simulink model "lab3_e1"  (R2016a)
settings: Solver=VariableStepAuto  StartTime=0.0  StopTime=50  RelTol=1e-3
values from neighbouring files (symbols this model uses):
  C_D = H'    [lab3_sumup.m]
  G_D = G'    [lab3_sumup.m]
  H_D = C'    [lab3_sumup.m]
  L_db = acker(G_D, H_D, [p0, p1])    [lab3_sumup.m]
  L_ndb = acker(G_D, H_D, [p0, p1])    [lab3_sumup.m]
  Ts = 0.75    [lab3_sumup.m]
  x = [0 0.3]'    [lab3_sumup.m]
settings Model: Creator=Helvins  LastModifiedBy=Helvins

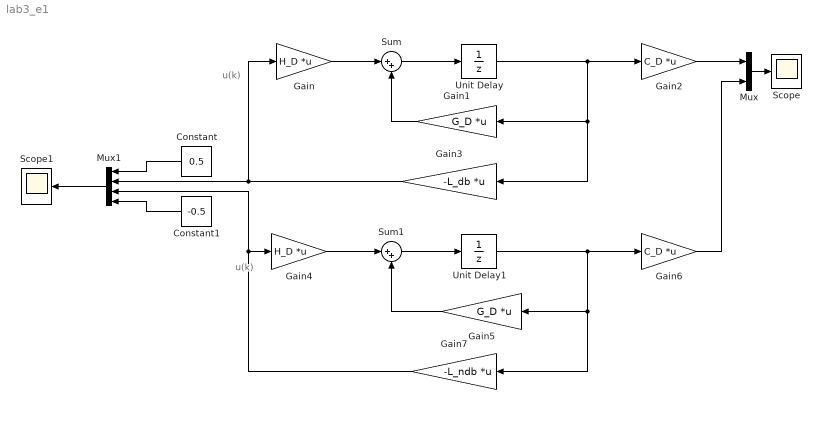
== system lab3_e1 ==
  note: u(k)
  note: u(k)
  Constant : Constant  Value=0.5
  Constant1 : Constant  Value=-0.5
  Gain : Gain  Gain=H_D  Multiplication=Matrix(K*u)
  Gain1 : Gain  Gain=G_D  Multiplication=Matrix(K*u)
  Gain2 : Gain  Gain=C_D  Multiplication=Matrix(K*u)
  Gain3 : Gain  Gain=-L_db  Multiplication=Matrix(K*u)
  Gain4 : Gain  Gain=H_D  Multiplication=Matrix(K*u)
  Gain5 : Gain  Gain=G_D  Multiplication=Matrix(K*u)
  Gain6 : Gain  Gain=C_D  Multiplication=Matrix(K*u)
  Gain7 : Gain  Gain=-L_ndb  Multiplication=Matrix(K*u)
  Mux : Mux  Inputs=2
  Mux1 : Mux
  Scope : Scope
  Scope1 : Scope
  Sum : Sum  Inputs=|++
  Sum1 : Sum  Inputs=|++
  Unit Delay : UnitDelay  InitialCondition=[x(1);x(2)]  SampleTime=Ts
  Unit Delay1 : UnitDelay  InitialCondition=[x(1);x(2)]  SampleTime=Ts
  wires:
  Gain/1 -> Sum/1
  Gain1/1 -> Sum/2
  Sum/1 -> Unit Delay/1
  Unit Delay/1 -> Gain1/1, Gain3/1, Gain2/1
  Gain4/1 -> Sum1/1
  Gain5/1 -> Sum1/2
  Sum1/1 -> Unit Delay1/1
  Unit Delay1/1 -> Gain5/1, Gain7/1, Gain6/1
  Gain7/1 -> Mux1/3, Gain4/1
  Gain2/1 -> Mux/1
  Mux/1 -> Scope/1
  Gain6/1 -> Mux/2
  Mux1/1 -> Scope1/1
  Gain3/1 -> Mux1/2, Gain/1
  Constant/1 -> Mux1/1
  Constant1/1 -> Mux1/4
